simulink model "ques10"  (R2021a)
settings: Solver=VariableStepAuto  StartTime=0.0  StopTime=5  RelTol=1e-3
libraries: simulink x1
settings Model: Creator=AVM  LastModifiedBy=AVM

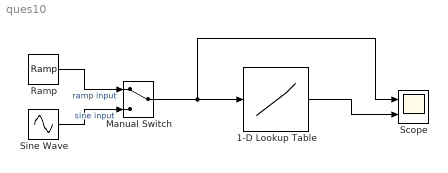
== system ques10 ==
  1-D Lookup Table : Lookup_n-D  NumberOfTableDimensions=1  BreakpointsForDimension1=[0 0.1 0.2 0.3 0.4 0.6 0.8 1.0 1.2 1.4 1.6 1.8 2.0 2.2 2.4]  Table=[0 0 0 0 0.5 1 2 3 5 7.5 10 15 20 25 30]  InternalRulePriority=Speed  RndMeth=Simplest  InputSameDT=on
  Manual Switch : ManualSwitch
  Ramp : simulink/Sources/Ramp  slope=1  start=0  InitialOutput=0
  Scope : Scope  NumInputPorts=2
  Sine Wave : Sin  SampleTime=0
  wires:
  1-D Lookup Table/1 -> Scope/2
  Ramp/1 -> Manual Switch/1  "ramp input"
  Sine Wave/1 -> Manual Switch/2  "sine input"
  Manual Switch/1 -> 1-D Lookup Table/1, Scope/1
